simulink model "FunctionalArch"  (R2025a)
settings: Solver=VariableStepAuto  StartTime=0.0  StopTime=10.0  RelTol=1e-3
settings Model: Creator=mfussi  LastModifiedBy=mfussi

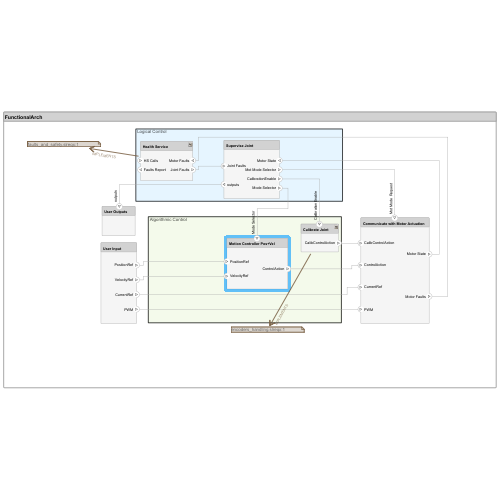
[thumbnail: Simulink's stored preview of the top-level diagram]
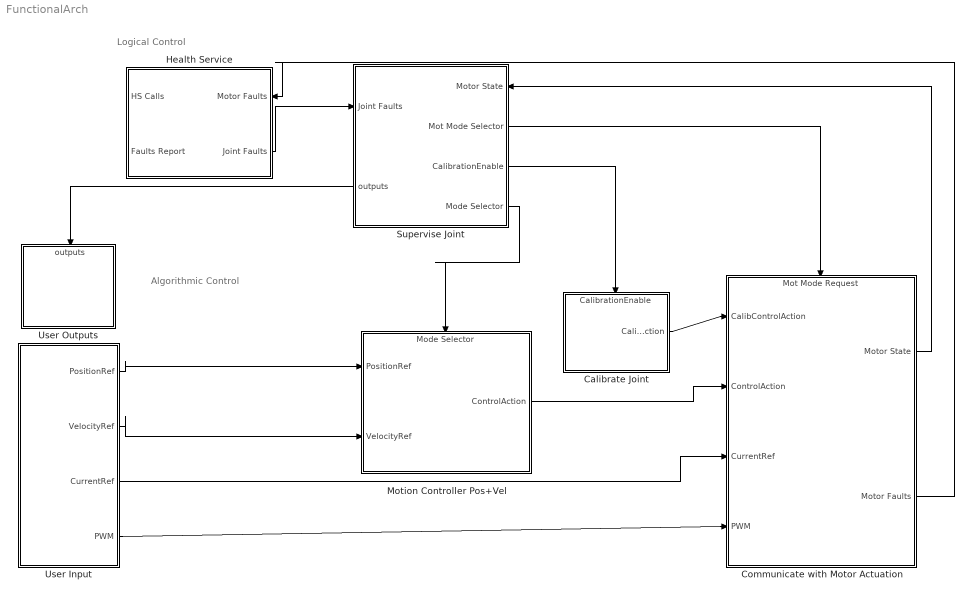
== system FunctionalArch ==
  note: Algorithmic Control
  note: Logical Control
  Calibrate Joint : Subsystem
      settings: PortSchema="{\"entries\":[{\"content\":{\"headerSize\":26,\"margin\":15,\"minimumSpacing\":25,\"sides\":[{\"content\":{},\"type\":\"ConnectorPlacement.EquallySpacedRectSide\",\"uuid\":\"01a9f67f-de41-4770-8c99-b8ecc5be53ce\"},{\"content\":{\"connectorIds\":[\"Out1\"],\"side\":\"RIGHT\"},\"type\":\"ConnectorPlacement.EquallySpacedRectSide\",\"uuid\":\"bf951eb2-be85-4331-ab1b-e1ec4c58de10\"},{\"content\":{\"connectorIds\":[\"In1\"],\"side\":\"TOP\"},\"type\":\"ConnectorPlacement.EquallySpacedRectSide\",\"uuid\":\"bda0090a-3dbc-4c35-be89-fb46a9401bc0\"},{\"content\":{\"side\":\"BOTTOM\"},\"type\":\"ConnectorPlacement.EquallySpacedRectSide\",\"uuid\":\"ec3dea10-cab4-440e-89eb-654eef2537c3\"}]},\"type\":\"ConnectorPlacement.EquallySpacedConnector\",\"uuid\":\"c83d3565-87fc-4d8e-ad9f-6c471e7c3840\"}],\"packageUris\":[\"http://schema.mathworks.com/mf0/Connector/R2020b\"],\"version\":\"1.0\"}"
  Communicate with Motor Actuation : Subsystem
      settings: PortSchema="{\"entries\":[{\"content\":{\"headerSize\":26,\"margin\":15,\"minimumSpacing\":25,\"sides\":[{\"content\":{\"connectorIds\":[\"In2\",\"In5\",\"In3\",\"In4\"]},\"type\":\"ConnectorPlacement.EquallySpacedRectSide\",\"uuid\":\"01a9f67f-de41-4770-8c99-b8ecc5be53ce\"},{\"content\":{\"connectorIds\":[\"Out2\",\"Out1\"],\"side\":\"RIGHT\"},\"type\":\"ConnectorPlacement.EquallySpacedRectSide\",\"uuid\":\"bf951eb2-be85-4331-ab1b-e1ec4c58de10\"},{\"content\":{\"connectorIds\":[\"In1\"],\"side\":\"TOP\"},\"type\":\"ConnectorPlacement.EquallySpacedRectSide\",\"uuid\":\"bda0090a-3dbc-4c35-be89-fb46a9401bc0\"},{\"content\":{\"side\":\"BOTTOM\"},\"type\":\"ConnectorPlacement.EquallySpacedRectSide\",\"uuid\":\"f7131699-3452-4999-9aaf-c54facf454ce\"}]},\"type\":\"ConnectorPlacement.EquallySpacedConnector\",\"uuid\":\"c83d3565-87fc-4d8e-ad9f-6c471e7c3840\"}],\"packageUris\":[\"http://schema.mathworks.com/mf0/Connector/R2020b\"],\"version\":\"1.0\"}"
  Health Service : Subsystem
      settings: PortSchema="{\"entries\":[{\"content\":{\"headerSize\":26,\"margin\":15,\"minimumSpacing\":25,\"sides\":[{\"content\":{\"connectorIds\":[\"In1\",\"Out1\"]},\"type\":\"ConnectorPlacement.EquallySpacedRectSide\",\"uuid\":\"be32944e-0d92-4c67-8eee-e106a8eb1edc\"},{\"content\":{\"connectorIds\":[\"In2\",\"Out2\"],\"side\":\"RIGHT\"},\"type\":\"ConnectorPlacement.EquallySpacedRectSide\",\"uuid\":\"3707551c-772d-48c3-8ee1-f2bbd92bf62d\"},{\"content\":{\"side\":\"TOP\"},\"type\":\"ConnectorPlacement.EquallySpacedRectSide\",\"uuid\":\"07c2d3b8-9fbc-4fed-8874-66ed938b2614\"},{\"content\":{\"side\":\"BOTTOM\"},\"type\":\"ConnectorPlacement.EquallySpacedRectSide\",\"uuid\":\"7a02bec9-749c-4b15-a822-29076ce65808\"}]},\"type\":\"ConnectorPlacement.EquallySpacedConnector\",\"uuid\":\"db3d3912-df38-43cf-94bf-5e9c07c8dbe9\"}],\"packageUris\":[\"http://schema.mathworks.com/mf0/Connector/R2020b\"],\"version\":\"1.0\"}"
  Motion Controller Pos+Vel : Subsystem
      settings: PortSchema="{\"entries\":[{\"content\":{\"headerSize\":26,\"margin\":15,\"minimumSpacing\":25,\"sides\":[{\"content\":{\"connectorIds\":[\"In2\",\"In3\"]},\"type\":\"ConnectorPlacement.EquallySpacedRectSide\",\"uuid\":\"242ec434-dfb9-46ff-b691-34edcc6b7cb4\"},{\"content\":{\"connectorIds\":[\"Out1\"],\"side\":\"RIGHT\"},\"type\":\"ConnectorPlacement.EquallySpacedRectSide\",\"uuid\":\"d1d7208e-7a5d-43b6-a69a-b0871ec22dc1\"},{\"content\":{\"connectorIds\":[\"In1\"],\"side\":\"TOP\"},\"type\":\"ConnectorPlacement.EquallySpacedRectSide\",\"uuid\":\"aa25ce41-c3c5-42be-848d-4335a5c5eaca\"}]},\"type\":\"ConnectorPlacement.EquallySpacedConnector\",\"uuid\":\"3938d3e3-056e-4ec6-b0b0-11c959115c92\"}],\"packageUris\":[\"http://schema.mathworks.com/mf0/Connector/R2020b\"],\"version\":\"1.0\"}"
  Supervise Joint : Subsystem
      settings: PortSchema="{\"entries\":[{\"content\":{\"headerSize\":26,\"margin\":15,\"minimumSpacing\":25,\"sides\":[{\"content\":{\"connectorIds\":[\"In2\",\"Out4\"]},\"type\":\"ConnectorPlacement.EquallySpacedRectSide\",\"uuid\":\"8e6109ac-b489-4864-8b2b-7ebf0beccfe4\"},{\"content\":{\"connectorIds\":[\"In1\",\"Out3\",\"Out2\",\"Out1\"],\"side\":\"RIGHT\"},\"type\":\"ConnectorPlacement.EquallySpacedRectSide\",\"uuid\":\"71828a7e-6b05-4f57-abc1-6f865453b9f6\"},{\"content\":{\"side\":\"TOP\"},\"type\":\"ConnectorPlacement.EquallySpacedRectSide\",\"uuid\":\"bfeeaaf9-6170-4b48-807f-b679c72692dc\"},{\"content\":{\"side\":\"BOTTOM\"},\"type\":\"ConnectorPlacement.EquallySpacedRectSide\",\"uuid\":\"8d96d7f2-73a1-4d5a-99fb-90680abef3dc\"}]},\"type\":\"ConnectorPlacement.EquallySpacedConnector\",\"uuid\":\"352ed8e9-1880-4bea-97e7-a2aba6f573a0\"}],\"packageUris\":[\"http://schema.mathworks.com/mf0/Connector/R2020b\"],\"version\":\"1.0\"}"
  User Input : Subsystem
      settings: PortSchema="{\"entries\":[{\"content\":{\"headerSize\":26,\"margin\":15,\"minimumSpacing\":25,\"sides\":[{\"content\":{},\"type\":\"ConnectorPlacement.EquallySpacedRectSide\",\"uuid\":\"a711e3b8-e43e-480a-948b-1eb4056efe2d\"},{\"content\":{\"connectorIds\":[\"Out1\",\"Out2\",\"Out3\",\"Out4\"],\"side\":\"RIGHT\"},\"type\":\"ConnectorPlacement.EquallySpacedRectSide\",\"uuid\":\"3f041336-352a-4053-9c0c-fa1eb8499c1b\"},{\"content\":{\"side\":\"TOP\"},\"type\":\"ConnectorPlacement.EquallySpacedRectSide\",\"uuid\":\"a6c29d4b-a30c-4c55-990f-cc7c775b3131\"},{\"content\":{\"side\":\"BOTTOM\"},\"type\":\"ConnectorPlacement.EquallySpacedRectSide\",\"uuid\":\"c443904e-a4fe-467e-a78f-6e3cebde01b7\"}]},\"type\":\"ConnectorPlacement.EquallySpacedConnector\",\"uuid\":\"e01ca2db-d7ea-4d7e-8660-1651b0279799\"}],\"packageUris\":[\"http://schema.mathworks.com/mf0/Connector/R2020b\"],\"version\":\"1.0\"}"
  User Outputs : Subsystem
      settings: PortSchema="{\"entries\":[{\"content\":{\"headerSize\":26,\"margin\":15,\"minimumSpacing\":25,\"sides\":[{\"content\":{},\"type\":\"ConnectorPlacement.EquallySpacedRectSide\",\"uuid\":\"631d8a47-b3f2-4e31-a63d-0648e710a315\"},{\"content\":{\"side\":\"RIGHT\"},\"type\":\"ConnectorPlacement.EquallySpacedRectSide\",\"uuid\":\"0d0ad518-2986-41ed-bfd4-93cc12acf9fd\"},{\"content\":{\"connectorIds\":[\"In1\"],\"side\":\"TOP\"},\"type\":\"ConnectorPlacement.EquallySpacedRectSide\",\"uuid\":\"1ac8e51d-d00a-42d6-bf71-b1f045e3befc\"}]},\"type\":\"ConnectorPlacement.EquallySpacedConnector\",\"uuid\":\"6fde844f-6155-4562-bf7c-07c1612c594e\"}],\"packageUris\":[\"http://schema.mathworks.com/mf0/Connector/R2020b\"],\"version\":\"1.0\"}"
  wires:
  Calibrate Joint/1(CalibControlAction) -> Communicate with Motor Actuation/2(CalibControlAction)
  Supervise Joint/2(CalibrationEnable) -> Calibrate Joint/1(CalibrationEnable)
  Supervise Joint/3(Mot Mode Selector) -> Communicate with Motor Actuation/1(Mot Mode Request)
  Communicate with Motor Actuation/1(Motor Faults) -> Health Service/2(Motor Faults)
  Health Service/2(Joint Faults) -> Supervise Joint/2(Joint Faults)
  Communicate with Motor Actuation/2(Motor State) -> Supervise Joint/1(Motor State)
  User Input/3(CurrentRef) -> Communicate with Motor Actuation/3(CurrentRef)
  Supervise Joint/4(outputs) -> User Outputs/1(outputs)
  User Input/4(PWM) -> Communicate with Motor Actuation/4(PWM)
  Supervise Joint/1(Mode Selector) -> Motion Controller Pos+Vel/1(Mode Selector)
  User Input/1(PositionRef) -> Motion Controller Pos+Vel/2(PositionRef)
  User Input/2(VelocityRef) -> Motion Controller Pos+Vel/3(VelocityRef)
  Motion Controller Pos+Vel/1(ControlAction) -> Communicate with Motor Actuation/5(ControlAction)

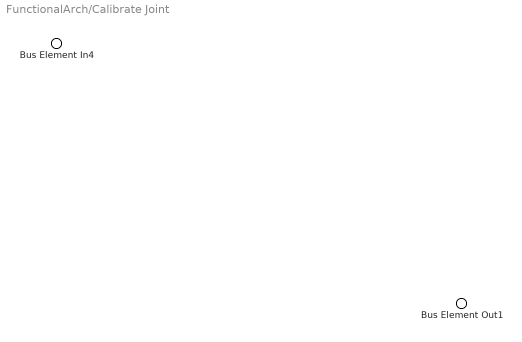
== system FunctionalArch/Calibrate Joint ==
  Bus Element In4 : Inport  PortName=CalibrationEnable
  Bus Element Out1 : Outport  PortName=CalibControlAction

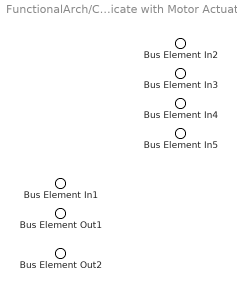
== system FunctionalArch/Communicate with Motor Actuation ==
  Bus Element In3 : Inport  PortName=Mot Mode Request
  Bus Element In2 : Inport  Port=2  PortName=CalibControlAction
  Bus Element In4 : Inport  Port=3  PortName=CurrentRef
  Bus Element In5 : Inport  Port=4  PortName=PWM
  Bus Element In1 : Inport  Port=5  PortName=ControlAction
  Bus Element Out1 : Outport  PortName=Motor Faults
  Bus Element Out2 : Outport  Port=2  PortName=Motor State

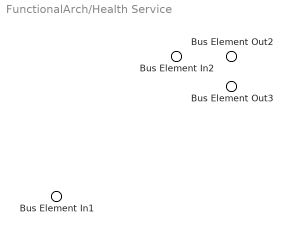
== system FunctionalArch/Health Service ==
  Bus Element In2 : Inport  PortName=HS Calls
  Bus Element In1 : Inport  Port=2  PortName=Motor Faults
  Bus Element Out3 : Outport  PortName=Faults Report
  Bus Element Out2 : Outport  Port=2  PortName=Joint Faults

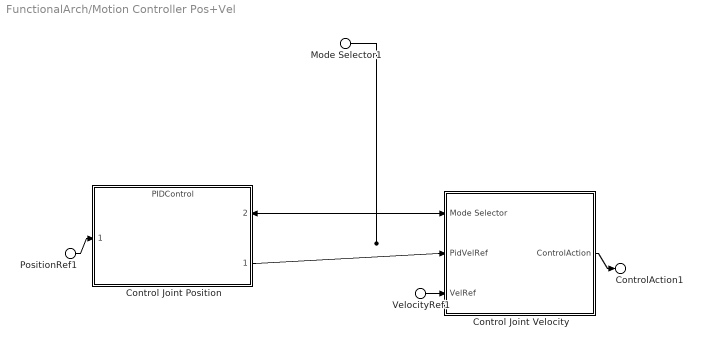
== system FunctionalArch/Motion Controller Pos+Vel ==
  Mode Selector1 : Inport  PortName=Mode Selector
  PositionRef1 : Inport  Port=2  PortName=PositionRef
  VelocityRef1 : Inport  Port=3  PortName=VelocityRef
  Control Joint Position : ModelReference  ModelNameDialog=PIDControl  SimulationMode=Normal  ModelReferenceVersion=1.19
      settings: PortSchema="{\"entries\":[{\"content\":{\"headerSize\":38,\"margin\":15,\"minimumSpacing\":25,\"sides\":[{\"content\":{\"connectorIds\":[\"In1\"]},\"type\":\"ConnectorPlacement.EquallySpacedRectSide\",\"uuid\":\"a6b52f4d-c0be-425e-a602-92486203cf1a\"},{\"content\":{\"connectorIds\":[\"In2\",\"Out1\"],\"side\":\"RIGHT\"},\"type\":\"ConnectorPlacement.EquallySpacedRectSide\",\"uuid\":\"97de3152-cc67-4140-b6b8-81845a876737\"},{\"content\":{\"side\":\"TOP\"},\"type\":\"ConnectorPlacement.EquallySpacedRectSide\",\"uuid\":\"ebc405a6-c557-4a2e-ab17-42ca9b397efe\"},{\"content\":{\"side\":\"BOTTOM\"},\"type\":\"ConnectorPlacement.EquallySpacedRectSide\",\"uuid\":\"fc9b133b-bd9a-4a39-bcaa-9d91c54c3b24\"}]},\"type\":\"ConnectorPlacement.EquallySpacedConnector\",\"uuid\":\"3652fe7f-5812-4192-9520-9c06c6702b26\"}],\"packageUris\":[\"http://schema.mathworks.com/mf0/Connector/R2020b\"],\"version\":\"1.0\"}"
  Control Joint Velocity : Subsystem
      settings: PortSchema="{\"entries\":[{\"content\":{\"headerSize\":26,\"margin\":15,\"minimumSpacing\":25,\"sides\":[{\"content\":{\"connectorIds\":[\"In1\",\"In3\",\"In2\"]},\"type\":\"ConnectorPlacement.EquallySpacedRectSide\",\"uuid\":\"be32944e-0d92-4c67-8eee-e106a8eb1edc\"},{\"content\":{\"connectorIds\":[\"Out1\"],\"side\":\"RIGHT\"},\"type\":\"ConnectorPlacement.EquallySpacedRectSide\",\"uuid\":\"3707551c-772d-48c3-8ee1-f2bbd92bf62d\"},{\"content\":{\"side\":\"TOP\"},\"type\":\"ConnectorPlacement.EquallySpacedRectSide\",\"uuid\":\"07c2d3b8-9fbc-4fed-8874-66ed938b2614\"},{\"content\":{\"side\":\"BOTTOM\"},\"type\":\"ConnectorPlacement.EquallySpacedRectSide\",\"uuid\":\"65f52ead-8a23-4c59-b5f1-2fdc368bd61c\"}]},\"type\":\"ConnectorPlacement.EquallySpacedConnector\",\"uuid\":\"db3d3912-df38-43cf-94bf-5e9c07c8dbe9\"}],\"packageUris\":[\"http://schema.mathworks.com/mf0/Connector/R2020b\"],\"version\":\"1.0\"}"
  ControlAction1 : Outport  PortName=ControlAction
  wires:
  Control Joint Position/1 -> Control Joint Velocity/3(PidVelRef)
  Control Joint Velocity/1(ControlAction) -> ControlAction1/1
  Mode Selector1/1 -> Control Joint Velocity/1(Mode Selector), Control Joint Position/2
  VelocityRef1/1 -> Control Joint Velocity/2(VelRef)
  PositionRef1/1 -> Control Joint Position/1

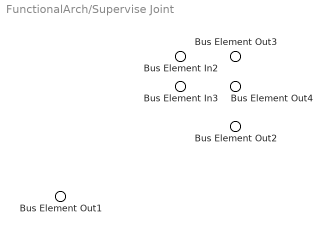
== system FunctionalArch/Supervise Joint ==
  Bus Element In3 : Inport  PortName=Motor State
  Bus Element In2 : Inport  Port=2  PortName=Joint Faults
  Bus Element Out1 : Outport  PortName=Mode Selector
  Bus Element Out3 : Outport  Port=2  PortName=CalibrationEnable
  Bus Element Out4 : Outport  Port=3  PortName=Mot Mode Selector
  Bus Element Out2 : Outport  Port=4  PortName=outputs

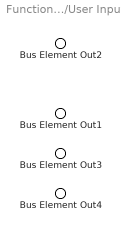
== system FunctionalArch/User Input ==
  Bus Element Out2 : Outport  PortName=PositionRef
  Bus Element Out1 : Outport  Port=2  PortName=VelocityRef
  Bus Element Out3 : Outport  Port=3  PortName=CurrentRef
  Bus Element Out4 : Outport  Port=4  PortName=PWM

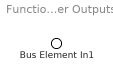
== system FunctionalArch/User Outputs ==
  Bus Element In1 : Inport  PortName=outputs

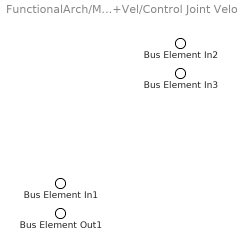
== system FunctionalArch/Motion Controller Pos+Vel/Control Joint Velocity ==
  Bus Element In2 : Inport  PortName=Mode Selector
  Bus Element In3 : Inport  Port=2  PortName=VelRef
  Bus Element In1 : Inport  Port=3  PortName=PidVelRef
  Bus Element Out1 : Outport  PortName=ControlAction
